simulink model "simu"  (R2025a)
settings: Solver=ode4  StartTime=0.0  StopTime=150  FixedStep=0.01  RelTol=1e-3
settings Model: Creator=lenovo  LastModifiedBy=lenovo
settings DataIOCC: ReturnWorkspaceOutputs=off

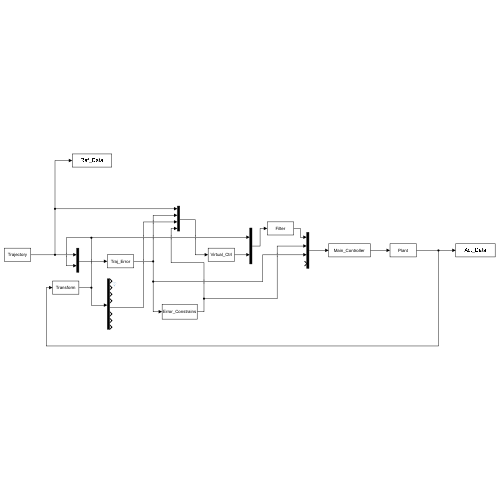
[thumbnail: Simulink's stored preview of the top-level diagram]
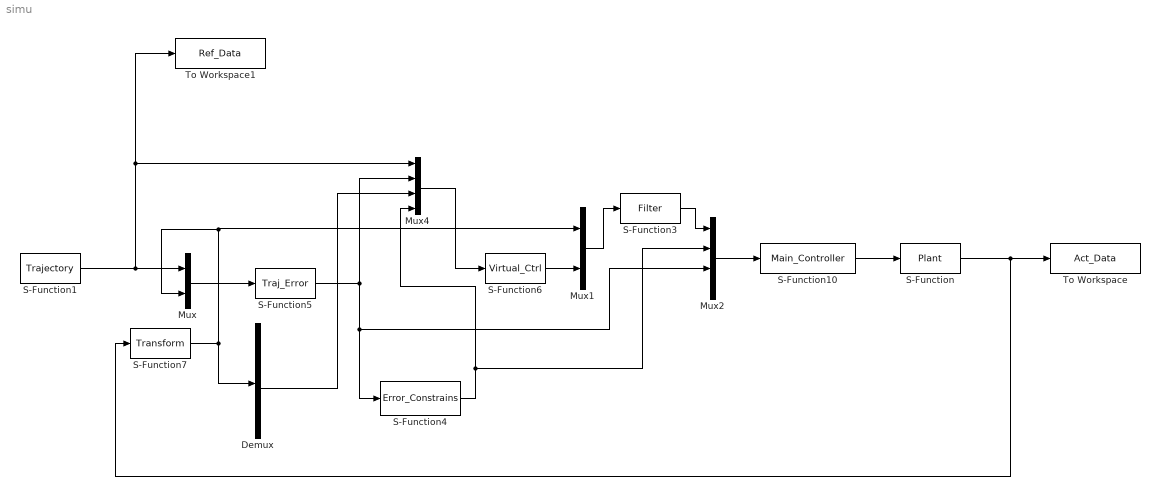
== system simu ==
  Demux : Demux  Outputs=8
  Mux : Mux  Inputs=2
  Mux1 : Mux  Inputs=2
  Mux2 : Mux
  Mux4 : Mux
  S-Function : S-Function  FunctionName=Plant  SFunctionDeploymentMode=off  EnableBusSupport=off
  S-Function1 : S-Function  FunctionName=Trajectory  SFunctionDeploymentMode=off  EnableBusSupport=off
  S-Function10 : S-Function  FunctionName=Main_Controller  SFunctionDeploymentMode=off  EnableBusSupport=off
  S-Function3 : S-Function  FunctionName=Filter  SFunctionDeploymentMode=off  EnableBusSupport=off
  S-Function4 : S-Function  FunctionName=Error_Constrains  SFunctionDeploymentMode=off  EnableBusSupport=off
  S-Function5 : S-Function  FunctionName=Traj_Error  SFunctionDeploymentMode=off  EnableBusSupport=off
  S-Function6 : S-Function  FunctionName=Virtual_Ctrl  SFunctionDeploymentMode=off  EnableBusSupport=off
  S-Function7 : S-Function  FunctionName=Transform  SFunctionDeploymentMode=off  EnableBusSupport=off
  To Workspace : ToWorkspace  VariableName=Act_Data  SaveFormat=Timeseries  SampleTime=-1
  To Workspace1 : ToWorkspace  VariableName=Ref_Data  SaveFormat=Timeseries  SampleTime=-1
  wires:
  S-Function5/1 -> Mux4/2, S-Function4/1, Mux2/3
  S-Function1/1 -> Mux/1, Mux4/1, To Workspace1/1
  S-Function7/1 -> Demux/1, Mux1/1, Mux/2
  Mux/1 -> S-Function5/1
  Mux1/1 -> S-Function3/1
  S-Function6/1 -> Mux1/2
  S-Function3/1 -> Mux2/1
  Mux2/1 -> S-Function10/1
  S-Function10/1 -> S-Function/1
  S-Function4/1 -> Mux4/4, Mux2/2
  Demux/5 -> Mux4/3
  Mux4/1 -> S-Function6/1
  S-Function/1 -> To Workspace/1, S-Function7/1
